simulink library "simetranss"  (R2024b)
settings: Solver=VariableStepAuto  StartTime=0.0  StopTime=10.0  RelTol=1e-3
PostLoadFcn:
  | Ts=1e-6
InitFcn:
  | Ts=1e-6
undefined symbols (not defined in the file): C, C_601, C_603, C_606, CC, Csnu, Csnubber, DiscIntNeverNeededParam, DPL, DPL1ph, FluxTable, ft2km, gcbh, h, Half, Imap2, L, L_601, L_603, L_606, Lbase, LpejoSw, Newton, R_601, R_603, R_606, Raphson, ResistanceM, Roff, Ron, RotorAngles, Rsnu, Rsnubber, Rt4, SampleTime, simetran, sps, sps_rtmsupport, StatorCurrents, T_2wind_ratio, T_Lpu, T_Lpu_pri, T_Rpu, T_Rpu_pri, T_Vpri, T_Vpri_15comp, T_Vsec, Ti, Ts_Power, Z, Zbase, Zm
libraries: fl_lib x248, ee_lib x146, nesl_utility x122, $bdroot x29, simulink x15, eeGeneralControl x2, spsStairGeneratorLib x2, artemis x1
(part 8 of 12)

== system simetranss/Power converters/Switching Function Interpolating 2-level inverter ==
  g : Inport
  Constant1 : Constant  Value=0
  Constant9 : Constant  Value=0
  Controlled Current Source1 : fl_lib/Electrical/Electrical Sources/Controlled Current Source
  Controlled Voltage Source : fl_lib/Electrical/Electrical Sources/Controlled Voltage Source
  Current Sensor : fl_lib/Electrical/Electrical Sensors/Current Sensor
  Demux1 : Demux  Outputs=2
  Fcn : Fcn  Expr=1-u
  PS-Simulink Converter : nesl_utility/PS-Simulink Converter  PhysicalDomain=network_engine_domain  SubClassName=ps_output  LeftPortType=input  RightPortType=output  PseudoPeriodic=off  Frequencies=[]  VectorFormat=inherit  Unit=inherit  AffineConversion=off
  PS-Simulink Converter1 : nesl_utility/PS-Simulink Converter  PhysicalDomain=network_engine_domain  SubClassName=ps_output  LeftPortType=input  RightPortType=output  PseudoPeriodic=off  Frequencies=[]  VectorFormat=inherit  Unit=inherit  AffineConversion=off
  Simulink-PS Converter : nesl_utility/Simulink-PS Converter  PhysicalDomain=network_engine_domain  SubClassName=ps_input  LeftPortType=input  RightPortType=output  PseudoPeriodic=off  Frequencies=[]  NoiseDistribution=none  NoiseParameters=[]  Unit=1  AffineConversion=off  FilteringAndDerivatives=provide  SimscapeFilterOrder=1  InputFilterTimeConstant=0.001  UdotUserProvided=0
  Simulink-PS Converter1 : nesl_utility/Simulink-PS Converter  PhysicalDomain=network_engine_domain  SubClassName=ps_input  LeftPortType=input  RightPortType=output  PseudoPeriodic=off  Frequencies=[]  NoiseDistribution=none  NoiseParameters=[]  Unit=1  AffineConversion=off  FilteringAndDerivatives=provide  SimscapeFilterOrder=1  InputFilterTimeConstant=0.001  UdotUserProvided=0
  Simulink-PS Converter2 : nesl_utility/Simulink-PS Converter  PhysicalDomain=network_engine_domain  SubClassName=ps_input  LeftPortType=input  RightPortType=output  PseudoPeriodic=off  Frequencies=[]  NoiseDistribution=none  NoiseParameters=[]  Unit=1  AffineConversion=off  FilteringAndDerivatives=provide  SimscapeFilterOrder=1  InputFilterTimeConstant=0.001  UdotUserProvided=0
  Switch : fl_lib/Electrical/Electrical Elements/Switch  R_closed=Ron Ohm  G_open=1e-5 1/Ohm  Threshold=0.5  i_specify=off  i_priority=None  i=0 A  i_nominal_specify=off  i_nominal_value=1  i_nominal_unit=A  v_specify=off  v_priority=None  v=0 V  v_nominal_specify=off  v_nominal_value=1  v_nominal_unit=V
  Switch1 : Switch  Threshold=0.5  SaturateOnIntegerOverflow=off  InputSameDT=off
  Switch4 : Switch  Threshold=0.5  SaturateOnIntegerOverflow=off  InputSameDT=off
  Unit Delay : UnitDelay  SampleTime=Ts  HasFrameUpgradeWarning=on
  Unit Delay1 : UnitDelay  SampleTime=Ts  HasFrameUpgradeWarning=on
  Voltage Sensor : fl_lib/Electrical/Electrical Sensors/Voltage Sensor
  ctrl1 : Subsystem
  lowthy : Subsystem
  upthy : Subsystem
  A : PMIOPort  Side=Left
  Dc+ : PMIOPort  Port=2  Side=Right
  Dc- : PMIOPort  Port=3  Side=Right
  wires:
  ctrl1/3(sw) -> [sw], Switch4/2, Switch1/2
  ctrl1/1(Idc) -> Switch1/1
  Switch1/1 -> Simulink-PS Converter/1
  Constant1/1 -> Switch1/3
  ctrl1/2(Vac) -> Switch4/1
  Constant9/1 -> Switch4/3
  Switch4/1 -> Simulink-PS Converter1/1
  Unit Delay1/1 -> ctrl1/3(Iac)
  Unit Delay/1 -> ctrl1/4(Vdc)
  Fcn/1 -> upthy/1(g), lowthy/1(g)
  [sw] -> Fcn/1
  [sw] -> Simulink-PS Converter2/1
  PS-Simulink Converter1/1 -> Unit Delay/1
  PS-Simulink Converter/1 -> lowthy/2(i), upthy/2("i "), Unit Delay1/1
  Demux1/1 -> ctrl1/1(g)
  Demux1/2 -> ctrl1/2(g1)
  g/1 -> Demux1/1
  connections:
  Switch/LConn1 -- Current Sensor/LConn1
  Controlled Voltage Source/LConn1 -- Switch/RConn2
  Current Sensor/RConn2 -- lowthy/RConn1 -- upthy/LConn1 -- A/RConn1
  PS-Simulink Converter1/LConn1 -- Voltage Sensor/RConn1
  upthy/RConn1 -- Dc+/RConn1 -- Voltage Sensor/LConn1 -- Controlled Current Source1/RConn2
  lowthy/LConn1 -- Voltage Sensor/RConn2 -- Controlled Voltage Source/RConn2 -- Controlled Current Source1/LConn1 -- Dc-/RConn1
  Simulink-PS Converter1/RConn1 -- Controlled Voltage Source/RConn1
  PS-Simulink Converter/LConn1 -- Current Sensor/RConn1
  Simulink-PS Converter/RConn1 -- Controlled Current Source1/RConn1
  Simulink-PS Converter2/RConn1 -- Switch/RConn1

== system simetranss/Switches/MATE 3ph Breaker ==
  C4 : Constant  Value=External
  Circuit Breaker : ee_lib/Switches & Breakers/Circuit Breaker  R_closed=BreakerResistance Ohm  G_open=1/Roff 1/Ohm  threshold=0.5 V  breaker_behavior=ee.enum.switches.breakerBehavior.zeroCrossingEnable
      settings: InternalSimscapePortConfiguration="{\"Bottom\":[],\"Left\":[{\"id\":\"vT\",\"label\":\"vT\",\"type\":\"input\"},{\"id\":\"p1\",\"label\":\"\",\"type\":\"foundation.electrical.electrical\"}],\"Right\":[{\"id\":\"p2\",\"label\":\"\",\"type\":\"foundation.electrical.electrical\"}],\"Top\":[]}"
  Circuit Breaker1 : ee_lib/Switches & Breakers/Circuit Breaker  R_closed=BreakerResistance Ohm  G_open=1/Roff 1/Ohm  threshold=0.5 V  breaker_behavior=ee.enum.switches.breakerBehavior.zeroCrossingEnable
      settings: InternalSimscapePortConfiguration="{\"Bottom\":[],\"Left\":[{\"id\":\"vT\",\"label\":\"vT\",\"type\":\"input\"},{\"id\":\"p1\",\"label\":\"\",\"type\":\"foundation.electrical.electrical\"}],\"Right\":[{\"id\":\"p2\",\"label\":\"\",\"type\":\"foundation.electrical.electrical\"}],\"Top\":[]}"
  Circuit Breaker2 : ee_lib/Switches & Breakers/Circuit Breaker  R_closed=BreakerResistance Ohm  G_open=1/Roff 1/Ohm  threshold=0.5 V  breaker_behavior=ee.enum.switches.breakerBehavior.zeroCrossingEnable
      settings: InternalSimscapePortConfiguration="{\"Bottom\":[],\"Left\":[{\"id\":\"vT\",\"label\":\"vT\",\"type\":\"input\"},{\"id\":\"p1\",\"label\":\"\",\"type\":\"foundation.electrical.electrical\"}],\"Right\":[{\"id\":\"p2\",\"label\":\"\",\"type\":\"foundation.electrical.electrical\"}],\"Top\":[]}"
  Constant1 : Constant  Value=SwitchA
  Constant2 : Constant  Value=SwitchB
  Constant3 : Constant  Value=SwitchC
  Constant5 : Constant  Value=InitialState
  Fcn : Fcn  Expr=1-u
  Fcn1 : Fcn  Expr=1-u
  Fcn2 : Fcn  Expr=1-u
  Phase Splitter1 : ee_lib/Connectors & References/Phase Splitter
  Phase Splitter2 : ee_lib/Connectors & References/Phase Splitter
  RCsnubber : Subsystem  Commented=on
  Simulink-PS Converter : nesl_utility/Simulink-PS Converter  PhysicalDomain=network_engine_domain  SubClassName=ps_input  LeftPortType=input  RightPortType=output  PseudoPeriodic=off  Frequencies=[]  NoiseDistribution=none  NoiseParameters=[]  Unit=1  AffineConversion=off  FilteringAndDerivatives=provide  SimscapeFilterOrder=1  InputFilterTimeConstant=0.001  UdotUserProvided=0
  Simulink-PS Converter1 : nesl_utility/Simulink-PS Converter  PhysicalDomain=network_engine_domain  SubClassName=ps_input  LeftPortType=input  RightPortType=output  PseudoPeriodic=off  Frequencies=[]  NoiseDistribution=none  NoiseParameters=[]  Unit=1  AffineConversion=off  FilteringAndDerivatives=provide  SimscapeFilterOrder=1  InputFilterTimeConstant=0.001  UdotUserProvided=0
  Simulink-PS Converter2 : nesl_utility/Simulink-PS Converter  PhysicalDomain=network_engine_domain  SubClassName=ps_input  LeftPortType=input  RightPortType=output  PseudoPeriodic=off  Frequencies=[]  NoiseDistribution=none  NoiseParameters=[]  Unit=1  AffineConversion=off  FilteringAndDerivatives=provide  SimscapeFilterOrder=1  InputFilterTimeConstant=0.001  UdotUserProvided=0
  Stair Generator : spsStairGeneratorLib/Stair Generator  t=Switch_Times  e=SwitchStates  Ts=Ts
  Switch : Switch  Threshold=0.5  ZeroCross=off  SaturateOnIntegerOverflow=off
  Switch1 : Switch  Threshold=0.5  ZeroCross=off  SaturateOnIntegerOverflow=off
  Switch2 : Switch  Threshold=0.5  ZeroCross=off  SaturateOnIntegerOverflow=off
  Switch3 : Switch  Threshold=0.5  ZeroCross=off  SaturateOnIntegerOverflow=off  InputSameDT=off
  com : Constant
  abc : PMIOPort  Side=Left
  ABC : PMIOPort  Port=2  Side=Right
  wires:
  Switch3/1 -> Switch2/1, Switch1/1, Switch/1
  Constant1/1 -> Switch/2
  Switch/1 -> Fcn/1
  Constant3/1 -> Switch2/2
  Switch2/1 -> Fcn2/1
  Constant2/1 -> Switch1/2
  Switch1/1 -> Fcn1/1
  C4/1 -> Switch3/2
  com/1 -> Switch3/1
  Stair Generator/1 -> Switch3/3
  Constant5/1 -> Switch/3, Switch1/3, Switch2/3
  Fcn/1 -> Simulink-PS Converter/1
  Fcn1/1 -> Simulink-PS Converter1/1
  Fcn2/1 -> Simulink-PS Converter2/1
  connections:
  Circuit Breaker/LConn1 -- Simulink-PS Converter/RConn1
  RCsnubber/LConn2 -- Phase Splitter2/RConn2 -- Circuit Breaker1/LConn2
  Phase Splitter2/LConn1 -- abc/RConn1
  Circuit Breaker/LConn2 -- Phase Splitter2/RConn1 -- RCsnubber/LConn3
  RCsnubber/LConn1 -- Phase Splitter2/RConn3 -- Circuit Breaker2/LConn2
  Circuit Breaker1/LConn1 -- Simulink-PS Converter1/RConn1
  Circuit Breaker2/LConn1 -- Simulink-PS Converter2/RConn1
  Phase Splitter1/LConn1 -- ABC/RConn1
  Phase Splitter1/RConn1 -- Circuit Breaker/RConn1 -- RCsnubber/RConn1
  RCsnubber/RConn2 -- Phase Splitter1/RConn2 -- Circuit Breaker1/RConn1
  RCsnubber/RConn3 -- Phase Splitter1/RConn3 -- Circuit Breaker2/RConn1

== system simetranss/Switches/MATE Breaker ==
  C4 : Constant  Value=External
  Circuit Breaker : ee_lib/Switches & Breakers/Circuit Breaker  R_closed=BreakerResistance Ohm  G_open=1/Roff 1/Ohm  threshold=0.5 V  breaker_behavior=ee.enum.switches.breakerBehavior.zeroCrossingEnable
      settings: InternalSimscapePortConfiguration="{\"Bottom\":[],\"Left\":[{\"id\":\"vT\",\"label\":\"vT\",\"type\":\"input\"},{\"id\":\"p1\",\"label\":\"\",\"type\":\"foundation.electrical.electrical\"}],\"Right\":[{\"id\":\"p2\",\"label\":\"\",\"type\":\"foundation.electrical.electrical\"}],\"Top\":[]}"
  Constant1 : Constant  Value=SwitchA
  Constant5 : Constant  Value=InitialState
  Fcn : Fcn  Expr=1-u
  RCsnubber : Subsystem  Commented=on
  Simulink-PS Converter : nesl_utility/Simulink-PS Converter  PhysicalDomain=network_engine_domain  SubClassName=ps_input  LeftPortType=input  RightPortType=output  PseudoPeriodic=off  Frequencies=[]  NoiseDistribution=none  NoiseParameters=[]  Unit=1  AffineConversion=off  FilteringAndDerivatives=provide  SimscapeFilterOrder=1  InputFilterTimeConstant=0.001  UdotUserProvided=0
  Stair Generator : spsStairGeneratorLib/Stair Generator  t=Switch_Times  e=SwitchStates  Ts=Ts
  Switch : Switch  Threshold=0.5  ZeroCross=off  SaturateOnIntegerOverflow=off
  Switch3 : Switch  Threshold=0.5  ZeroCross=off  SaturateOnIntegerOverflow=off  InputSameDT=off
  com : Constant
  a : PMIOPort  Side=Left
  A : PMIOPort  Port=2  Side=Right
  wires:
  Fcn/1 -> Simulink-PS Converter/1
  Constant5/1 -> Switch/3
  Stair Generator/1 -> Switch3/3
  com/1 -> Switch3/1
  C4/1 -> Switch3/2
  Switch/1 -> Fcn/1
  Constant1/1 -> Switch/2
  Switch3/1 -> Switch/1
  connections:
  Circuit Breaker/RConn1 -- RCsnubber/RConn1 -- A/RConn1
  Circuit Breaker/LConn2 -- RCsnubber/LConn1 -- a/RConn1
  Circuit Breaker/LConn1 -- Simulink-PS Converter/RConn1

== system simetranss/Usefulls/Event Timer ==
  Repeating Sequence : simulink/Sources/Repeating Sequence  rep_seq_t=st  rep_seq_y=sw
  Repeating Sequence1 : simulink/Sources/Repeating Sequence  Commented=on  rep_seq_t="[0    0.2000    0.2001    0.4000    0.4001    0.6000    2.0000]"  rep_seq_y=|
      | [     1     1     0     0     1     1     1
      | ]
  RTE : Outport  VectorParamsAs1DForOutWhenUnconnected=off
  wires:
  Repeating Sequence/1 -> RTE/1

== system simetranss/Usefulls/ModelInitialization ==

== system simetranss/FPGA/MATE 2-level inverter backup/Pejovic L//C switch2 ==
  gate : Inport
  Xin : Inport  Port=2
  Bus Creator : BusCreator  Inputs=2
  Controlled Current Source : fl_lib/Electrical/Electrical Sources/Controlled Current Source
  Current Sensor : fl_lib/Electrical/Electrical Sensors/Current Sensor
  Gain : Gain  Gain=-1
  Gain1 : Gain  Gain=1/Rsw
  Gain2 : Gain
  PS-Simulink Converter1 : nesl_utility/PS-Simulink Converter  PhysicalDomain=network_engine_domain  SubClassName=ps_output  LeftPortType=input  RightPortType=output  PseudoPeriodic=off  Frequencies=[]  VectorFormat=inherit  Unit=inherit  AffineConversion=off
  PS-Simulink Converter2 : nesl_utility/PS-Simulink Converter  PhysicalDomain=network_engine_domain  SubClassName=ps_output  LeftPortType=input  RightPortType=output  PseudoPeriodic=off  Frequencies=[]  VectorFormat=inherit  Unit=inherit  AffineConversion=off
  Relational Operator : RelationalOperator  Operator=~=  OutDataTypeStr=boolean  RndMeth=Simplest  InputSameDT=off
  Resistor : fl_lib/Electrical/Electrical Elements/Resistor  R=Rsw Ohm  i_specify=off  i_priority=None  i=0 A  i_nominal_specify=off  i_nominal_value=1  i_nominal_unit=A  v_specify=off  v_priority=None  v=0 V  v_nominal_specify=off  v_nominal_value=1  v_nominal_unit=V
  Simulink-PS Converter1 : nesl_utility/Simulink-PS Converter  PhysicalDomain=network_engine_domain  SubClassName=ps_input  LeftPortType=input  RightPortType=output  PseudoPeriodic=off  Frequencies=[]  NoiseDistribution=none  NoiseParameters=[]  Unit=1  AffineConversion=off  FilteringAndDerivatives=provide  SimscapeFilterOrder=1  InputFilterTimeConstant=0.001  UdotUserProvided=0
  Switch : Switch  Criteria=u2 > Threshold  Threshold=0.5  SaturateOnIntegerOverflow=off  InputSameDT=off
  Switch1 : Switch  Criteria=u2 > Threshold  Threshold=0.5  SaturateOnIntegerOverflow=off  InputSameDT=off
  Switch2 : Switch  Criteria=u2 > Threshold  Threshold=0.5  SaturateOnIntegerOverflow=off  InputSameDT=off
  Unit Delay : UnitDelay  SampleTime=Ts  HasFrameUpgradeWarning=on
  Unit Delay1 : UnitDelay  SampleTime=Ts  HasFrameUpgradeWarning=on
  Unit Delay2 : UnitDelay  SampleTime=Ts  HasFrameUpgradeWarning=on
  Voltage Sensor : fl_lib/Electrical/Electrical Sensors/Voltage Sensor
  +V : PMIOPort  Side=Left
  -V : PMIOPort  Port=2  Side=Right
  meas : Outport
  Xout : Outport  Port=2
  wires:
  PS-Simulink Converter2/1 -> [Vsw]
  PS-Simulink Converter1/1 -> [Isw]
  Switch/1 -> Unit Delay/1
  [Isw] -> Gain/1
  Gain/1 -> Switch/1
  [Vsw] -> Gain1/1
  Gain1/1 -> Switch2/3, Switch/3
  [Ihist] -> Simulink-PS Converter1/1
  [Isw] -> Bus Creator/2  "Switch current (A)"
  [Vsw] -> Bus Creator/1  "Switch voltage (V)"
  Bus Creator/1 -> meas/1
  Switch1/1 -> [Ihist]
  Unit Delay/1 -> Switch1/3
  Xin/1 -> Switch1/1
  Unit Delay1/1 -> Relational Operator/1
  Relational Operator/1 -> Switch1/2
  Gain2/1 -> Switch2/1
  [Isw] -> Gain2/1
  Switch2/1 -> Unit Delay2/1
  gate/1 -> Switch2/2, Relational Operator/2, Unit Delay1/1, Switch/2
  Unit Delay2/1 -> Xout/1
  connections:
  Resistor/RConn1 -- Voltage Sensor/RConn2 -- -V/RConn1 -- Controlled Current Source/RConn2
  Current Sensor/RConn2 -- Voltage Sensor/LConn1 -- Resistor/LConn1 -- Controlled Current Source/LConn1
  PS-Simulink Converter2/LConn1 -- Voltage Sensor/RConn1
  Controlled Current Source/RConn1 -- Simulink-PS Converter1/RConn1
  +V/RConn1 -- Current Sensor/LConn1
  Current Sensor/RConn1 -- PS-Simulink Converter1/LConn1

== system simetranss/FPGA/MATE 2-level inverter backup/Pejovic L//C switch3 ==
  gate : Inport
  Xin : Inport  Port=2
  Bus Creator : BusCreator  Inputs=2
  Controlled Current Source : fl_lib/Electrical/Electrical Sources/Controlled Current Source
  Current Sensor : fl_lib/Electrical/Electrical Sensors/Current Sensor
  Gain : Gain  Gain=-1
  Gain1 : Gain  Gain=1/Rsw
  Gain2 : Gain
  PS-Simulink Converter1 : nesl_utility/PS-Simulink Converter  PhysicalDomain=network_engine_domain  SubClassName=ps_output  LeftPortType=input  RightPortType=output  PseudoPeriodic=off  Frequencies=[]  VectorFormat=inherit  Unit=inherit  AffineConversion=off
  PS-Simulink Converter2 : nesl_utility/PS-Simulink Converter  PhysicalDomain=network_engine_domain  SubClassName=ps_output  LeftPortType=input  RightPortType=output  PseudoPeriodic=off  Frequencies=[]  VectorFormat=inherit  Unit=inherit  AffineConversion=off
  Relational Operator : RelationalOperator  Operator=~=  OutDataTypeStr=boolean  RndMeth=Simplest  InputSameDT=off
  Resistor : fl_lib/Electrical/Electrical Elements/Resistor  R=Rsw Ohm  i_specify=off  i_priority=None  i=0 A  i_nominal_specify=off  i_nominal_value=1  i_nominal_unit=A  v_specify=off  v_priority=None  v=0 V  v_nominal_specify=off  v_nominal_value=1  v_nominal_unit=V
  Simulink-PS Converter1 : nesl_utility/Simulink-PS Converter  PhysicalDomain=network_engine_domain  SubClassName=ps_input  LeftPortType=input  RightPortType=output  PseudoPeriodic=off  Frequencies=[]  NoiseDistribution=none  NoiseParameters=[]  Unit=1  AffineConversion=off  FilteringAndDerivatives=provide  SimscapeFilterOrder=1  InputFilterTimeConstant=0.001  UdotUserProvided=0
  Switch : Switch  Criteria=u2 > Threshold  Threshold=0.5  SaturateOnIntegerOverflow=off  InputSameDT=off
  Switch1 : Switch  Criteria=u2 > Threshold  Threshold=0.5  SaturateOnIntegerOverflow=off  InputSameDT=off
  Switch2 : Switch  Criteria=u2 > Threshold  Threshold=0.5  SaturateOnIntegerOverflow=off  InputSameDT=off
  Unit Delay : UnitDelay  SampleTime=Ts  HasFrameUpgradeWarning=on
  Unit Delay1 : UnitDelay  SampleTime=Ts  HasFrameUpgradeWarning=on
  Unit Delay2 : UnitDelay  SampleTime=Ts  HasFrameUpgradeWarning=on
  Voltage Sensor : fl_lib/Electrical/Electrical Sensors/Voltage Sensor
  +V : PMIOPort  Side=Left
  -V : PMIOPort  Port=2  Side=Right
  meas : Outport
  Xout : Outport  Port=2
  wires:
  Relational Operator/1 -> Switch1/2
  Unit Delay1/1 -> Relational Operator/1
  Xin/1 -> Switch1/1
  Unit Delay/1 -> Switch1/3
  Switch1/1 -> [Ihist]
  Bus Creator/1 -> meas/1
  [Vsw] -> Bus Creator/1  "Switch voltage (V)"
  [Isw] -> Bus Creator/2  "Switch current (A)"
  [Ihist] -> Simulink-PS Converter1/1
  [Vsw] -> Gain1/1
  Gain/1 -> Switch/1
  [Isw] -> Gain/1
  Switch/1 -> Unit Delay/1
  PS-Simulink Converter1/1 -> [Isw]
  PS-Simulink Converter2/1 -> [Vsw]
  Gain2/1 -> Switch2/1
  [Isw] -> Gain2/1
  gate/1 -> Switch/2, Switch2/2, Unit Delay1/1, Relational Operator/2
  Switch2/1 -> Unit Delay2/1
  Gain1/1 -> Switch/3, Switch2/3
  Unit Delay2/1 -> Xout/1
  connections:
  Current Sensor/RConn1 -- PS-Simulink Converter1/LConn1
  +V/RConn1 -- Current Sensor/LConn1
  Controlled Current Source/RConn1 -- Simulink-PS Converter1/RConn1
  PS-Simulink Converter2/LConn1 -- Voltage Sensor/RConn1
  Controlled Current Source/LConn1 -- Resistor/LConn1 -- Voltage Sensor/LConn1 -- Current Sensor/RConn2
  Controlled Current Source/RConn2 -- -V/RConn1 -- Voltage Sensor/RConn2 -- Resistor/RConn1

== system simetranss/FPGA/MATE 2level_Inverter SwitchingFunction(3ph)/SW ==
  note: 1 = no pulse
      | 0 = pulse
  note: 0 == mode diode
      | 0 ~= mode pulse
  note: 1 = mode HighZ
      | 0 = mode pulse or diode
  gu : Inport
  gl : Inport  Port=2
  Vdc : Inport  Port=3
  Iac : Inport  Port=4
  Compare To Zero : simulink/Logic and Bit Operations/Compare To Zero  relop=>  OutDataTypeStr=uint8
  Constant : Constant
  Dead Zone : DeadZone  LowerValue=-min_charge  UpperValue=min_charge
  Divide : Product  Inputs=3
  Divide1 : Product
  Divide3 : Product
  Gain1 : Gain  Gain=Gp
  INT : Subsystem
  Logical Operator{1,4..5,8} (4 alike) : Logic  AllPortsSameDT=off  OutDataTypeStr=boolean
  Logical Operator{2..3,7,9} (4 alike) : Logic  Operator=NOT  AllPortsSameDT=off  OutDataTypeStr=boolean
  Logical Operator6 : Logic  Operator=OR  Inputs=3  AllPortsSameDT=off  OutDataTypeStr=boolean
  Logical_Not1 : Constant  Value=0  SampleTime=-1
  Relational Operator1 : RelationalOperator  Operator=>  OutDataTypeStr=boolean  InputSameDT=off
  Sum : Sum  Inputs=|++
  Sum1 : Sum  Inputs=--+
  Sum2 : Sum  Inputs=|++
  Sum6 : Sum  Inputs=-+  InputSameDT=on  SaturateOnIntegerOverflow=on  SampleTime=Ts  OutDataTypeStr=Inherit: Same as first input
  Switch : Switch  Criteria=u2 > Threshold  SaturateOnIntegerOverflow=off  InputSameDT=off
  Switch1 : Switch  Criteria=u2 ~= 0  SaturateOnIntegerOverflow=off  InputSameDT=off
  Switch2 : Switch  Criteria=u2 ~= 0  Threshold=0.5  SaturateOnIntegerOverflow=off  InputSameDT=off
  Switch3 : Switch  Criteria=u2 ~= 0  Threshold=0.5  SaturateOnIntegerOverflow=off  InputSameDT=off
  Unit Delay1 : UnitDelay  SampleTime=Ts  HasFrameUpgradeWarning=on
  Unit Delay2 : UnitDelay  SampleTime=Ts  HasFrameUpgradeWarning=on
  Idc : Outport  VectorParamsAs1DForOutWhenUnconnected=off
  Vac : Outport  Port=2  VectorParamsAs1DForOutWhenUnconnected=off
  wires:
  Unit Delay2/1 -> Logical Operator8/2, Logical Operator9/1
  Unit Delay1/1 -> [Vout]
  Switch3/1 -> Switch2/3
  Dead Zone/1 -> Switch3/1
  Divide/1 -> Dead Zone/1, Switch2/1, Switch3/3
  Switch2/1 -> Idc/1
  Switch/1 -> Switch1/1
  Logical Operator6/1 -> Logical Operator1/2, Unit Delay2/1
  Divide1/1 -> Switch1/3
  Sum2/1 -> Divide/2, Divide1/2
  gu/1 -> Sum1/1, Sum2/1, Sum/1
  Sum/1 -> Logical Operator2/1
  Compare To Zero/1 -> Logical Operator5/1, Logical Operator4/1, Logical Operator7/1
  Vdc/1 -> [Vin], Divide1/1
  [Vout] -> Relational Operator1/2
  Logical Operator2/1 -> Logical Operator1/1, Switch3/2
  Logical Operator3/1 -> Divide/3
  [Vin] -> Relational Operator1/1
  gl/1 -> Sum/2, Sum1/2
  Logical Operator7/1 -> Divide3/1
  Relational Operator1/1 -> Logical Operator5/2, Logical Operator8/1
  Logical Operator9/1 -> Logical Operator4/2
  Logical Operator4/1 -> Logical Operator6/1
  Logical Operator5/1 -> Logical Operator6/2
  Logical Operator8/1 -> Logical Operator6/3
  Constant/1 -> Sum1/3
  Sum1/1 -> Divide3/2
  Divide3/1 -> Sum2/2
  Switch1/1 -> Vac/1, Unit Delay1/1
  [Vout] -> INT/2(Initial)
  INT/1(u_p) -> Sum6/2
  Sum6/1 -> Switch/2, Switch/1
  Logical_Not1/1 -> Switch/3
  Logical Operator1/1 -> Switch2/2, Switch1/2, INT/3(en), Logical Operator3/1
  Gain1/1 -> Sum6/1
  Iac/1 -> Divide/1, Compare To Zero/1, INT/1(u), Gain1/1

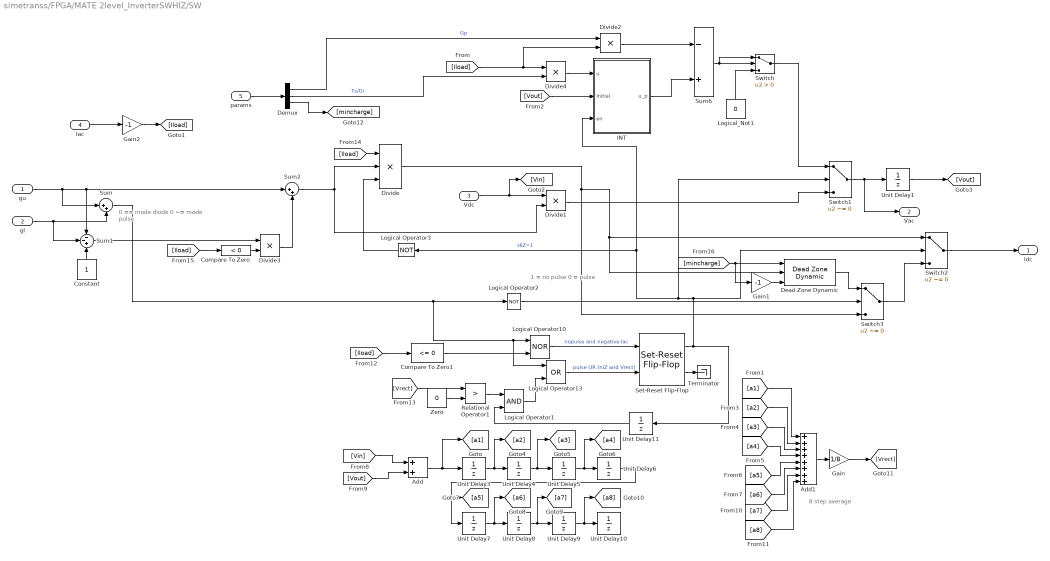
== system simetranss/FPGA/MATE 2level_InverterSWHIZ/SW ==
  note: 8 step average
  note: 1 = no pulse
      | 0 = pulse
  note: 0 == mode diode
      | 0 ~= mode pulse
  gu : Inport
  gl : Inport  Port=2
  Vdc : Inport  Port=3
  Iac : Inport  Port=4
  params : Inport  Port=5
  Add : Sum
  Add1 : Sum  Inputs=8
  Compare To Zero : simulink/Logic and Bit Operations/Compare To Zero  relop=<  OutDataTypeStr=uint8
  Compare To Zero1 : simulink/Logic and Bit Operations/Compare To Zero  relop=<=  OutDataTypeStr=uint8
  Constant : Constant
  Dead Zone Dynamic : simulink/Discontinuities/Dead Zone Dynamic
  Demux : Demux  Outputs=3
  Divide : Product  Inputs=3
  Divide{1..4} (4 alike) : Product
  Gain : Gain  Gain=1/8
  Gain1 : Gain  Gain=-1
  Gain2 : Gain  Gain=-1
  INT : Subsystem
  Logical Operator1 : Logic  AllPortsSameDT=off  OutDataTypeStr=boolean
  Logical Operator10 : Logic  Operator=NOR  AllPortsSameDT=off  OutDataTypeStr=boolean
  Logical Operator13 : Logic  Operator=OR  AllPortsSameDT=off  OutDataTypeStr=boolean
  Logical Operator2 : Logic  Operator=NOT  AllPortsSameDT=off  OutDataTypeStr=boolean
  Logical Operator3 : Logic  Operator=NOT  AllPortsSameDT=off  OutDataTypeStr=boolean
  Logical_Not1 : Constant  Value=0  SampleTime=-1
  Relational Operator1 : RelationalOperator  Operator=>  OutDataTypeStr=boolean  InputSameDT=off
  Set-Reset Flip-Flop : eeGeneralControl/Set-Reset Flip-Flop  LabelModeActiveChoice=Discrete  UndefState=Set  Q0=0  Ts=Ts
  Sum : Sum  Inputs=|++
  Sum1 : Sum  Inputs=--+
  Sum2 : Sum  Inputs=|++
  Sum6 : Sum  Inputs=-+  InputSameDT=on  SaturateOnIntegerOverflow=on  SampleTime=Ts  OutDataTypeStr=Inherit: Same as first input
  Switch : Switch  Criteria=u2 > Threshold  SaturateOnIntegerOverflow=off  InputSameDT=off
  Switch1 : Switch  Criteria=u2 ~= 0  SaturateOnIntegerOverflow=off  InputSameDT=off
  Switch2 : Switch  Criteria=u2 ~= 0  Threshold=0.5  SaturateOnIntegerOverflow=off  InputSameDT=off
  Switch3 : Switch  Criteria=u2 ~= 0  Threshold=0.5  SaturateOnIntegerOverflow=off  InputSameDT=off
  Terminator : Terminator
  Unit Delay{1,3..11} (10 alike) : UnitDelay  SampleTime=Ts  HasFrameUpgradeWarning=on
  Zero : Constant  Value=0  OutDataTypeStr=Inherit: Inherit via back propagation
  Idc : Outport  VectorParamsAs1DForOutWhenUnconnected=off
  Vac : Outport  Port=2  VectorParamsAs1DForOutWhenUnconnected=off
  wires:
  params/1 -> Demux/1
  Gain1/1 -> Dead Zone Dynamic/3
  [mincharge] -> Gain1/1, Dead Zone Dynamic/1
  Demux/3 -> [mincharge]
  Demux/2 -> Divide4/2  "Ts/Gi"
  Divide4/1 -> INT/1(u)
  Divide2/1 -> Sum6/1
  Demux/1 -> Divide2/1  "Gp"
  Gain2/1 -> [Iload]
  Sum1/1 -> Divide3/1
  Compare To Zero/1 -> Divide3/2
  [Iload] -> Compare To Zero/1
  [Iload] -> Divide/1
  [Iload] -> Divide2/2, Divide4/1
  Logical Operator1/1 -> Logical Operator13/2
  Logical Operator13/1 -> Set-Reset Flip-Flop/2  "pulse OR (hiZ and Vrect)"
  Unit Delay11/1 -> Logical Operator1/2
  Relational Operator1/1 -> Logical Operator1/1
  Zero/1 -> Relational Operator1/2
  [Vrect] -> Relational Operator1/1
  INT/1(u_p) -> Sum6/2
  Compare To Zero1/1 -> Logical Operator10/2
  [Iload] -> Compare To Zero1/1
  Gain/1 -> [Vrect]
  Add1/1 -> Gain/1
  [a1] -> Add1/1
  [a8] -> Add1/8
  [a2] -> Add1/2
  [a7] -> Add1/7
  [a6] -> Add1/6
  [a3] -> Add1/3
  [a5] -> Add1/5
  [a4] -> Add1/4
  Unit Delay9/1 -> Unit Delay10/1, [a8]
  Unit Delay8/1 -> Unit Delay9/1, [a7]
  Unit Delay7/1 -> Unit Delay8/1, [a6]
  Unit Delay6/1 -> Unit Delay7/1, [a5]
  Unit Delay5/1 -> Unit Delay6/1, [a4]
  Unit Delay4/1 -> Unit Delay5/1, [a3]
  Unit Delay3/1 -> Unit Delay4/1, [a2]
  Add/1 -> Unit Delay3/1, [a1]
  [Vout] -> Add/2
  [Vin] -> Add/1
  [Vout] -> INT/2(Initial)
  Logical Operator10/1 -> Set-Reset Flip-Flop/1  "nopulse and negative Iac"
  Unit Delay1/1 -> [Vout]
  Switch3/1 -> Switch2/3
  Dead Zone Dynamic/1 -> Switch3/1
  Divide/1 -> Switch2/1, Dead Zone Dynamic/2, Switch3/3
  Switch2/1 -> Idc/1
  Switch/1 -> Switch1/1
  Divide1/1 -> Switch1/3
  Sum2/1 -> Divide/2, Divide1/2
  gu/1 -> Sum1/1, Sum2/1, Sum/1
  Sum/1 -> Logical Operator2/1, Logical Operator10/1, Logical Operator13/1
  Vdc/1 -> [Vin], Divide1/1
  Logical Operator2/1 -> Switch3/2
  Logical Operator3/1 -> Divide/3
  gl/1 -> Sum/2, Sum1/2
  Constant/1 -> Sum1/3
  Divide3/1 -> Sum2/2
  Switch1/1 -> Vac/1, Unit Delay1/1
  Sum6/1 -> Switch/2, Switch/1
  Logical_Not1/1 -> Switch/3
  Set-Reset Flip-Flop/1 -> Unit Delay11/1, Switch2/2, Switch1/2, INT/3(en), Logical Operator3/1  "HiZ=1"
  Iac/1 -> Gain2/1
  Set-Reset Flip-Flop/2 -> Terminator/1

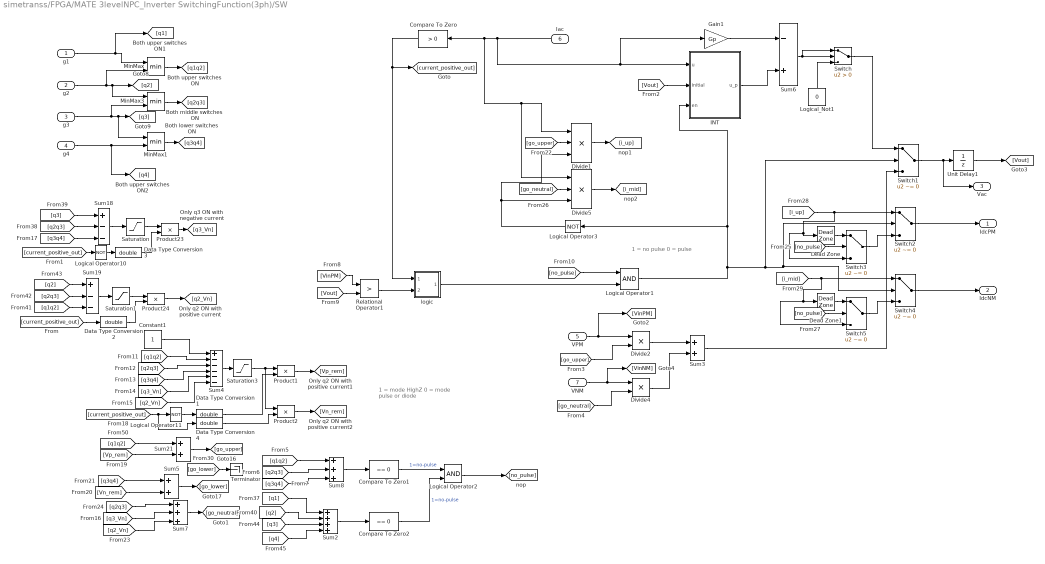
== system simetranss/FPGA/MATE 3levelNPC_Inverter SwitchingFunction(3ph)/SW ==
  note: 1 = no pulse
      | 0 = pulse
  note: 1 = mode HighZ
      | 0 = mode pulse or diode
  g1 : Inport
  g2 : Inport  Port=2
  g3 : Inport  Port=3
  g4 : Inport  Port=4
  VPM : Inport  Port=5
  Iac : Inport  Port=6
  VNM : Inport  Port=7
  Compare To Zero : simulink/Logic and Bit Operations/Compare To Zero  relop=>  OutDataTypeStr=uint8
  Compare To Zero1 : simulink/Logic and Bit Operations/Compare To Zero  relop===  OutDataTypeStr=uint8
  Compare To Zero2 : simulink/Logic and Bit Operations/Compare To Zero  relop===  OutDataTypeStr=uint8
  Constant1 : Constant
  Data Type Conversion{1..4} (4 alike) : DataTypeConversion  OutDataTypeStr=double
  Dead Zone : DeadZone  LowerValue=-min_charge  UpperValue=min_charge
  Dead Zone1 : DeadZone  LowerValue=-min_charge  UpperValue=min_charge
  Divide1 : Product  Inputs=3
  Divide2 : Product
  Divide4 : Product
  Divide5 : Product  Inputs=3
  Gain1 : Gain  Gain=Gp
  INT : Subsystem
  Logical Operator1 : Logic  AllPortsSameDT=off  OutDataTypeStr=boolean
  Logical Operator10 : Logic  Operator=NOT  AllPortsSameDT=off  OutDataTypeStr=boolean
  Logical Operator11 : Logic  Operator=NOT  AllPortsSameDT=off  OutDataTypeStr=boolean
  Logical Operator2 : Logic  AllPortsSameDT=off  OutDataTypeStr=boolean
  Logical Operator3 : Logic  Operator=NOT  AllPortsSameDT=off  OutDataTypeStr=boolean
  Logical_Not1 : Constant  Value=0  SampleTime=-1
  MinMax : MinMax  Inputs=2  InputSameDT=on  SaturateOnIntegerOverflow=on
  MinMax1 : MinMax  Inputs=2  InputSameDT=on  SaturateOnIntegerOverflow=on
  MinMax3 : MinMax  Inputs=2  InputSameDT=on  SaturateOnIntegerOverflow=on
  Product{1..2,23..24} (4 alike) : Product  InputSameDT=on  SaturateOnIntegerOverflow=on  OutDataTypeStr=Inherit: Same as first input
  Relational Operator1 : RelationalOperator  Operator=>  OutDataTypeStr=boolean  InputSameDT=off
  Saturation : Saturate  UpperLimit=1  LowerLimit=0
  Saturation1 : Saturate  UpperLimit=1  LowerLimit=0
  Saturation3 : Saturate  UpperLimit=1  LowerLimit=0
  Sum18 : Sum  Inputs=+--  InputSameDT=on  SaturateOnIntegerOverflow=on  OutDataTypeStr=Inherit: Same as first input
  Sum19 : Sum  Inputs=+--  InputSameDT=on  SaturateOnIntegerOverflow=on  OutDataTypeStr=Inherit: Same as first input
  Sum2 : Sum  Inputs=++++  InputSameDT=on  SaturateOnIntegerOverflow=on  OutDataTypeStr=Inherit: Same as first input
  Sum21 : Sum  InputSameDT=on  SaturateOnIntegerOverflow=on  OutDataTypeStr=Inherit: Same as first input
  Sum3 : Sum  InputSameDT=on  SaturateOnIntegerOverflow=on  OutDataTypeStr=Inherit: Same as first input
  Sum4 : Sum  Inputs=+-----  InputSameDT=on  SaturateOnIntegerOverflow=on  OutDataTypeStr=Inherit: Same as first input
  Sum5 : Sum  InputSameDT=on  SaturateOnIntegerOverflow=on  OutDataTypeStr=Inherit: Same as first input
  Sum6 : Sum  Inputs=-+  InputSameDT=on  SaturateOnIntegerOverflow=on  SampleTime=Ts  OutDataTypeStr=Inherit: Same as first input
  Sum7 : Sum  Inputs=+++  InputSameDT=on  SaturateOnIntegerOverflow=on  OutDataTypeStr=Inherit: Same as first input
  Sum8 : Sum  Inputs=+++  InputSameDT=on  SaturateOnIntegerOverflow=on  OutDataTypeStr=Inherit: Same as first input
  Switch : Switch  Criteria=u2 > Threshold  SaturateOnIntegerOverflow=off  InputSameDT=off
  Switch{1..5} (5 alike) : Switch  Criteria=u2 ~= 0  Threshold=0.5  SaturateOnIntegerOverflow=off  InputSameDT=off
  Terminator : Terminator
  Unit Delay1 : UnitDelay  SampleTime=Ts  HasFrameUpgradeWarning=on
  logic : Subsystem
  IdcPM : Outport  VectorParamsAs1DForOutWhenUnconnected=off
  IdcNM : Outport  Port=2  VectorParamsAs1DForOutWhenUnconnected=off
  Vac : Outport  Port=3  VectorParamsAs1DForOutWhenUnconnected=off
  wires:
  logic/1(Out1) -> Logical Operator1/2
  Relational Operator1/1 -> logic/2(In2)
  [go_lower] -> Terminator/1
  Switch1/1 -> Unit Delay1/1, Vac/1
  Logical Operator2/1 -> [no_pulse]
  Compare To Zero2/1 -> Logical Operator2/2  "1=no-pulse"
  Compare To Zero1/1 -> Logical Operator2/1  "1=no-pulse"
  Sum2/1 -> Compare To Zero2/1
  [q4] -> Sum2/4
  [q3] -> Sum2/3
  [q2] -> Sum2/2
  [q1] -> Sum2/1
  [Vout] -> INT/2(Initial)
  Unit Delay1/1 -> [Vout]
  Iac/1 -> Divide1/1, Divide5/1, Compare To Zero/1, INT/1(u), Gain1/1
  Switch/1 -> Switch1/1
  [q3q4] -> Sum8/3
  [q2q3] -> Sum8/2
  [q1q2] -> Sum8/1
  [i_mid] -> Switch4/1, Switch5/3, Dead Zone1/1
  [i_up] -> Switch2/1, Dead Zone/1, Switch3/3
  [no_pulse] -> Switch5/2
  [no_pulse] -> Switch3/2
  Divide5/1 -> [i_mid]
  [go_neutral] -> Divide5/2
  Switch4/1 -> IdcNM/1
  Dead Zone1/1 -> Switch5/1
  Switch5/1 -> Switch4/3
  [go_upper] -> Divide1/2
  Divide1/1 -> [i_up]
  Sum8/1 -> Compare To Zero1/1
  Divide4/1 -> Sum3/2
  Divide2/1 -> Sum3/1
  [go_neutral] -> Divide4/2
  VNM/1 -> Divide4/1, [VinNM]
  [go_upper] -> Divide2/2
  VPM/1 -> Divide2/1, [VinPM]
  [q2_Vn] -> Sum7/3
  Sum7/1 -> [go_neutral]
  [q3_Vn] -> Sum7/2
  [q2q3] -> Sum7/1
  [q3q4] -> Sum5/1
  [Vn_rem] -> Sum5/2
  [Vp_rem] -> Sum21/2
  Saturation3/1 -> Product1/1, Product2/1
  Data Type Conversion4/1 -> Product2/2
  Product2/1 -> [Vn_rem]
  Data Type Conversion1/1 -> Product1/2
  [current_positive_out] -> Logical Operator11/1, Data Type Conversion4/1
  Logical Operator11/1 -> Data Type Conversion1/1
  Sum4/1 -> Saturation3/1
  Product1/1 -> [Vp_rem]
  [q2_Vn] -> Sum4/6
  [q3_Vn] -> Sum4/5
  [q3q4] -> Sum4/4
  [q2q3] -> Sum4/3
  [q1q2] -> Sum4/2
  Constant1/1 -> Sum4/1
  Sum5/1 -> [go_lower]
  Sum21/1 -> [go_upper]
  [q1q2] -> Sum21/1
  Logical Operator10/1 -> Data Type Conversion3/1
  Data Type Conversion2/1 -> Product24/2
  [current_positive_out] -> Logical Operator10/1
  Sum19/1 -> Saturation1/1
  [q1q2] -> Sum19/3
  Product23/1 -> [q3_Vn]
  [current_positive_out] -> Data Type Conversion2/1
  Saturation/1 -> Product23/1
  Data Type Conversion3/1 -> Product23/2
  Saturation1/1 -> Product24/1
  [q2q3] -> Sum19/2
  Product24/1 -> [q2_Vn]
  [q2] -> Sum19/1
  Sum18/1 -> Saturation/1
  [q3q4] -> Sum18/3
  [q3] -> Sum18/1
  [q2q3] -> Sum18/2
  g4/1 -> MinMax1/2, [q4]
  g2/1 -> [q2], MinMax3/1, MinMax/2
  g3/1 -> MinMax3/2, [q3], MinMax1/1
  g1/1 -> MinMax/1, [q1]
  MinMax1/1 -> [q3q4]
  MinMax/1 -> [q1q2]
  MinMax3/1 -> [q2q3]
  Switch3/1 -> Switch2/3
  Dead Zone/1 -> Switch3/1
  Switch2/1 -> IdcPM/1
  Sum3/1 -> Switch1/3
  Compare To Zero/1 -> logic/1(In1), [current_positive_out]
  [Vout] -> Relational Operator1/2
  [no_pulse] -> Logical Operator1/1
  Logical Operator3/1 -> Divide5/3, Divide1/3
  [VinPM] -> Relational Operator1/1
  INT/1(u_p) -> Sum6/2
  Sum6/1 -> Switch/2, Switch/1
  Logical_Not1/1 -> Switch/3
  Logical Operator1/1 -> Switch2/2, Switch4/2, Switch1/2, Logical Operator3/1, INT/3(en)
  Gain1/1 -> Sum6/1

== system simetranss/Lines/Half-DPL/Simscape ==
  Electrical Reference1 : fl_lib/Electrical/Electrical Elements/Electrical Reference
  PS-S : nesl_utility/PS-Simulink Converter  PhysicalDomain=network_engine_domain  SubClassName=ps_output  LeftPortType=input  RightPortType=output  PseudoPeriodic=off  Frequencies=[]  VectorFormat=1-D array  Unit=V  AffineConversion=off
  Voltage Sensor : fl_lib/Electrical/Electrical Sensors/Voltage Sensor
  V : PMIOPort  Side=Left
  Out : Outport  VectorParamsAs1DForOutWhenUnconnected=off
  wires:
  PS-S/1 -> Out/1  "voltage"
  connections:
  PS-S/LConn1 -- Voltage Sensor/RConn1
  V/RConn1 -- Voltage Sensor/LConn1
  Electrical Reference1/LConn1 -- Voltage Sensor/RConn2

== system simetranss/Lines/Half-DPL/Simscape1 ==
  Electrical Reference1 : fl_lib/Electrical/Electrical Elements/Electrical Reference
  PS-S : nesl_utility/PS-Simulink Converter  PhysicalDomain=network_engine_domain  SubClassName=ps_output  LeftPortType=input  RightPortType=output  PseudoPeriodic=off  Frequencies=[]  VectorFormat=1-D array  Unit=V  AffineConversion=off
  Voltage Sensor : fl_lib/Electrical/Electrical Sensors/Voltage Sensor
  V : PMIOPort  Side=Left
  Out : Outport  VectorParamsAs1DForOutWhenUnconnected=off
  wires:
  PS-S/1 -> Out/1  "voltage"
  connections:
  Electrical Reference1/LConn1 -- Voltage Sensor/RConn2
  V/RConn1 -- Voltage Sensor/LConn1
  PS-S/LConn1 -- Voltage Sensor/RConn1

== system simetranss/Lines/Half-DPL/Simscape2 ==
  Electrical Reference1 : fl_lib/Electrical/Electrical Elements/Electrical Reference
  PS-S : nesl_utility/PS-Simulink Converter  PhysicalDomain=network_engine_domain  SubClassName=ps_output  LeftPortType=input  RightPortType=output  PseudoPeriodic=off  Frequencies=[]  VectorFormat=1-D array  Unit=V  AffineConversion=off
  Voltage Sensor : fl_lib/Electrical/Electrical Sensors/Voltage Sensor
  V : PMIOPort  Side=Left
  Out : Outport  VectorParamsAs1DForOutWhenUnconnected=off
  wires:
  PS-S/1 -> Out/1  "voltage"
  connections:
  PS-S/LConn1 -- Voltage Sensor/RConn1
  V/RConn1 -- Voltage Sensor/LConn1
  Electrical Reference1/LConn1 -- Voltage Sensor/RConn2

== system simetranss/Lines/Half-DPL/Voltage Source ==
  I : Inport
  Controlled Current Source1 : fl_lib/Electrical/Electrical Sources/Controlled Current Source
  Simulink-PS Converter : nesl_utility/Simulink-PS Converter  PhysicalDomain=network_engine_domain  SubClassName=ps_input  LeftPortType=input  RightPortType=output  PseudoPeriodic=off  Frequencies=[]  NoiseDistribution=none  NoiseParameters=[]  Unit=1  AffineConversion=off  FilteringAndDerivatives=zero  SimscapeFilterOrder=1  InputFilterTimeConstant=.001  UdotUserProvided=0
  + : PMIOPort  Side=Right
  - : PMIOPort  Port=2  Side=Right
  wires:
  I/1 -> Simulink-PS Converter/1
  connections:
  Controlled Current Source1/RConn1 -- Simulink-PS Converter/RConn1
  Controlled Current Source1/RConn2 -- -/RConn1
  Controlled Current Source1/LConn1 -- +/RConn1

== system simetranss/Lines/Half-DPL/Voltage Source1 ==
  I : Inport
  Controlled Current Source1 : fl_lib/Electrical/Electrical Sources/Controlled Current Source
  Simulink-PS Converter : nesl_utility/Simulink-PS Converter  PhysicalDomain=network_engine_domain  SubClassName=ps_input  LeftPortType=input  RightPortType=output  PseudoPeriodic=off  Frequencies=[]  NoiseDistribution=none  NoiseParameters=[]  Unit=1  AffineConversion=off  FilteringAndDerivatives=zero  SimscapeFilterOrder=1  InputFilterTimeConstant=.001  UdotUserProvided=0
  + : PMIOPort  Side=Right
  - : PMIOPort  Port=2  Side=Right
  wires:
  I/1 -> Simulink-PS Converter/1
  connections:
  Controlled Current Source1/LConn1 -- +/RConn1
  Controlled Current Source1/RConn2 -- -/RConn1
  Controlled Current Source1/RConn1 -- Simulink-PS Converter/RConn1

== system simetranss/Lines/Half-DPL/Voltage Source2 ==
  I : Inport
  Controlled Current Source1 : fl_lib/Electrical/Electrical Sources/Controlled Current Source
  Simulink-PS Converter : nesl_utility/Simulink-PS Converter  PhysicalDomain=network_engine_domain  SubClassName=ps_input  LeftPortType=input  RightPortType=output  PseudoPeriodic=off  Frequencies=[]  NoiseDistribution=none  NoiseParameters=[]  Unit=1  AffineConversion=off  FilteringAndDerivatives=zero  SimscapeFilterOrder=1  InputFilterTimeConstant=.001  UdotUserProvided=0
  + : PMIOPort  Side=Right
  - : PMIOPort  Port=2  Side=Right
  wires:
  I/1 -> Simulink-PS Converter/1
  connections:
  Controlled Current Source1/RConn1 -- Simulink-PS Converter/RConn1
  Controlled Current Source1/RConn2 -- -/RConn1
  Controlled Current Source1/LConn1 -- +/RConn1

== system simetranss/Lines/Half-DPL/dplmodel ==
  v : Inport
  hist_in : Inport  Port=2
  (1+h)/Z : Gain  Gain=(1+h)./(Zm+Rt4)  SaturateOnIntegerOverflow=on  OutDataTypeStr=Inherit: Same as input  ParamDataTypeStr=Inherit: Same as input
  Gain4 : Gain  Gain=(1+h)/2  SaturateOnIntegerOverflow=on  OutDataTypeStr=Inherit: Same as input  ParamDataTypeStr=Inherit: Same as input
  Gain6 : Gain  Gain=(1-h)/2  SaturateOnIntegerOverflow=on  OutDataTypeStr=Inherit: Same as input  ParamDataTypeStr=Inherit: Same as input
  Gain9 : Gain  Gain=h  SaturateOnIntegerOverflow=on  OutDataTypeStr=Inherit: Same as input  ParamDataTypeStr=Inherit: Same as input
  Matrix Gain1 : StateSpace  A=[]  B=[]  C=[]  D=K  InitialCondition=0  mask(Matrix Gain){K=Ti'}
      mask prompts: K "Gain matrix:"
      mask help: Matrix Gain.
      mask Help: Multiplies input vector by entered matrix to produce output vector (y=Au).
      mask Display: disp('K')
  Matrix Gain2 : StateSpace  A=[]  B=[]  C=[]  D=K  InitialCondition=0  mask(Matrix Gain){K=Ti}
      mask prompts: K "Gain matrix:"
      mask help: Matrix Gain.
      mask Help: Multiplies input vector by entered matrix to produce output vector (y=Au).
      mask Display: disp('K')
  Subsystem : Subsystem
  Sum1 : Sum  Inputs=-+  InputSameDT=on  SaturateOnIntegerOverflow=on  OutDataTypeStr=Inherit: Same as first input
  Sum3 : Sum  InputSameDT=on  SaturateOnIntegerOverflow=on  OutDataTypeStr=Inherit: Same as first input
  i : Outport  InitialOutput=0  VectorParamsAs1DForOutWhenUnconnected=off
  hist_out : Outport  Port=2  VectorParamsAs1DForOutWhenUnconnected=off
  wires:
  Matrix Gain2/1 -> i/1
  Matrix Gain1/1 -> (1+h)/Z/1
  Gain4/1 -> hist_out/1
  Gain9/1 -> Sum1/1
  Sum3/1 -> Matrix Gain2/1, Gain9/1
  (1+h)/Z/1 -> Sum1/2
  v/1 -> Matrix Gain1/1
  Gain6/1 -> Sum3/1
  hist_in/1 -> Sum3/2
  Subsystem/1(Out1) -> Gain4/1, Gain6/1
  Sum1/1 -> Subsystem/1(In1)

== system simetranss/Lines/Half-DPL1ph/Simscape ==
  Electrical Reference1 : fl_lib/Electrical/Electrical Elements/Electrical Reference
  PS-S : nesl_utility/PS-Simulink Converter  PhysicalDomain=network_engine_domain  SubClassName=ps_output  LeftPortType=input  RightPortType=output  PseudoPeriodic=off  Frequencies=[]  VectorFormat=1-D array  Unit=V  AffineConversion=off
  Voltage Sensor : fl_lib/Electrical/Electrical Sensors/Voltage Sensor
  V : PMIOPort  Side=Left
  Out : Outport  VectorParamsAs1DForOutWhenUnconnected=off
  wires:
  PS-S/1 -> Out/1  "voltage"
  connections:
  PS-S/LConn1 -- Voltage Sensor/RConn1
  V/RConn1 -- Voltage Sensor/LConn1
  Electrical Reference1/LConn1 -- Voltage Sensor/RConn2

== system simetranss/Lines/Half-DPL1ph/Voltage Source ==
  I : Inport
  Controlled Current Source1 : fl_lib/Electrical/Electrical Sources/Controlled Current Source
  Simulink-PS Converter : nesl_utility/Simulink-PS Converter  PhysicalDomain=network_engine_domain  SubClassName=ps_input  LeftPortType=input  RightPortType=output  PseudoPeriodic=off  Frequencies=[]  NoiseDistribution=none  NoiseParameters=[]  Unit=1  AffineConversion=off  FilteringAndDerivatives=zero  SimscapeFilterOrder=1  InputFilterTimeConstant=.001  UdotUserProvided=0
  + : PMIOPort  Side=Right
  - : PMIOPort  Port=2  Side=Right
  wires:
  I/1 -> Simulink-PS Converter/1
  connections:
  Controlled Current Source1/RConn1 -- Simulink-PS Converter/RConn1
  Controlled Current Source1/RConn2 -- -/RConn1
  Controlled Current Source1/LConn1 -- +/RConn1

== system simetranss/Lines/Half-DPL1ph/dplmodel ==
  v : Inport
  hist_in : Inport  Port=2
  (1+h)/Z : Gain  Gain=(1+h)./(Zm+Rt4)  SaturateOnIntegerOverflow=on  OutDataTypeStr=Inherit: Same as input  ParamDataTypeStr=Inherit: Same as input
  Gain4 : Gain  Gain=(1+h)/2  SaturateOnIntegerOverflow=on  OutDataTypeStr=Inherit: Same as input  ParamDataTypeStr=Inherit: Same as input
  Gain6 : Gain  Gain=(1-h)/2  SaturateOnIntegerOverflow=on  OutDataTypeStr=Inherit: Same as input  ParamDataTypeStr=Inherit: Same as input
  Gain9 : Gain  Gain=h  SaturateOnIntegerOverflow=on  OutDataTypeStr=Inherit: Same as input  ParamDataTypeStr=Inherit: Same as input
  Sum1 : Sum  Inputs=-+  InputSameDT=on  SaturateOnIntegerOverflow=on  OutDataTypeStr=Inherit: Same as first input
  Sum3 : Sum  InputSameDT=on  SaturateOnIntegerOverflow=on  OutDataTypeStr=Inherit: Same as first input
  derlay : Subsystem
  i : Outport  InitialOutput=0  VectorParamsAs1DForOutWhenUnconnected=off
  hist_out : Outport  Port=2  VectorParamsAs1DForOutWhenUnconnected=off
  wires:
  Sum3/1 -> i/1, Gain9/1
  v/1 -> (1+h)/Z/1
  Gain4/1 -> hist_out/1
  Gain9/1 -> Sum1/1
  (1+h)/Z/1 -> Sum1/2
  Gain6/1 -> Sum3/1
  hist_in/1 -> Sum3/2
  derlay/1(Out1) -> Gain4/1, Gain6/1
  Sum1/1 -> derlay/1(In1)

== system simetranss/Machines/MATE 6//4 SRM/Pos_sensor ==
  w : Inport
  Constant : Constant  Value=pi/2
  Discrete-Time Integrator : DiscreteIntegrator  InitialCondition=init_rotor_pos*pi/180  SampleTime=Ts  ICPrevOutput=DiscIntNeverNeededParam  ICPrevScaledInput=DiscIntNeverNeededParam
  Math Function : Math  Operator=mod  SignedPower=on
  angle : Outport  VectorParamsAs1DForOutWhenUnconnected=off
  wires:
  Math Function/1 -> angle/1
  Constant/1 -> Math Function/2
  Discrete-Time Integrator/1 -> Math Function/1
  w/1 -> Discrete-Time Integrator/1

== system simetranss/Machines/MATE Induction Machine/1 step prediction+2step averaging ==
  In1 : Inport
  Gain1 : Gain  Gain=0.5
  Gain2 : Gain  Gain=2
  Gain3 : Gain  Gain=-1
  Sum1 : Sum  SaturateOnIntegerOverflow=on
  Sum5 : Sum  SaturateOnIntegerOverflow=on
  Unit Delay1 : UnitDelay  SampleTime=Ts  HasFrameUpgradeWarning=on
  Out1 : Outport  VectorParamsAs1DForOutWhenUnconnected=off
  wires:
  In1/1 -> Sum1/2, Unit Delay1/1, Gain2/1
  Gain3/1 -> Sum5/2
  Gain2/1 -> Sum5/1
  Unit Delay1/1 -> Gain3/1
  Sum5/1 -> Sum1/1
  Sum1/1 -> Gain1/1
  Gain1/1 -> Out1/1

== system simetranss/Machines/MATE Induction Machine/Discretize (rotor Frame) ==
  Ac : Inport
  Bc : Inport  Port=2
  Cc : Inport  Port=3
  be : Inport  Port=4
  Enable : EnablePort
  2 euler factor : Gain  Gain=2  SaturateOnIntegerOverflow=on  OutDataTypeStr=Inherit: Same as input  ParamDataTypeStr=Inherit: Same as input
  Product1 : Product  Multiplication=Matrix(*)  SaturateOnIntegerOverflow=on  OutDataTypeStr=Inherit: Same as first input
  Product2 : Product  Multiplication=Matrix(*)  SaturateOnIntegerOverflow=on  OutDataTypeStr=Inherit: Same as first input
  Product4 : Product  Multiplication=Matrix(*)  SaturateOnIntegerOverflow=on  OutDataTypeStr=Inherit: Same as first input
  Sum1 : Sum  Inputs=+-  SaturateOnIntegerOverflow=on
  Sum2 : Sum  Inputs=2  SaturateOnIntegerOverflow=on
  Sum4 : Sum  Inputs=-+  SaturateOnIntegerOverflow=on
  Sum5 : Sum  SaturateOnIntegerOverflow=on
  Ts/2 : Gain  Gain=Ts/2  SaturateOnIntegerOverflow=on  OutDataTypeStr=Inherit: Same as input  ParamDataTypeStr=Inherit: Same as input
  inversion : Product  Inputs=/  Multiplication=Matrix(*)  RndMeth=Zero
  mult1 : Product
  mult2 : Product
  mult3 : Product
  trapeze has Ts/2 factor on B : Gain  Gain=Ts/2  SaturateOnIntegerOverflow=on  OutDataTypeStr=Inherit: Same as input  ParamDataTypeStr=Inherit: Same as input
  u1 : Constant
  u2 : Constant
  u3 : Constant  Value=eye(4,4)*Ts/2
  u5 : Constant  Value=eye(4,4)
  Ad : Outport  VectorParamsAs1DForOutWhenUnconnected=off
  Bd : Outport  Port=2  VectorParamsAs1DForOutWhenUnconnected=off
  Cd : Outport  Port=3  VectorParamsAs1DForOutWhenUnconnected=off
  bet : Outport  Port=4  VectorParamsAs1DForOutWhenUnconnected=off
  Bdspeedterm : Outport  Port=5  VectorParamsAs1DForOutWhenUnconnected=off
  wires:
  2 euler factor/1 -> Bdspeedterm/1
  Product2/1 -> 2 euler factor/1
  Sum2/1 -> mult2/2, mult1/2
  u3/1 -> Product2/2
  mult2/1 -> Product1/2
  Sum4/1 -> bet/1, mult3/2
  mult3/1 -> Sum5/2
  mult1/1 -> mult3/1, Sum1/2
  u1/1 -> Sum4/2
  be/1 -> Sum4/1, Sum2/2
  u2/1 -> Sum2/1
  Bc/1 -> trapeze has Ts/2 factor on B/1
  Cc/1 -> Cd/1
  inversion/1 -> Product4/1, Product2/1, Product1/1  "inv(I4-Ts/2*A)"
  trapeze has Ts/2 factor on B/1 -> mult2/1
  Ts/2/1 -> mult1/1
  Product4/1 -> Ad/1
  u5/1 -> Sum5/1, Sum1/1
  Sum5/1 -> Product4/2
  Product1/1 -> Bd/1
  Ac/1 -> Ts/2/1
  Sum1/1 -> inversion/1

== system simetranss/Machines/MATE Induction Machine/Discretize(fixed frame) ==
  Cc : Inport
  be : Inport  Port=2
  Enable : EnablePort
  Sum4 : Sum  Inputs=-+  SaturateOnIntegerOverflow=on
  u1 : Constant
  u3 : Constant  Value=Bdspeed
  u4 : Constant  Value=Ad
  u6 : Constant  Value=Bd
  Ad : Outport  VectorParamsAs1DForOutWhenUnconnected=off
  Bd : Outport  Port=2  VectorParamsAs1DForOutWhenUnconnected=off
  Cd : Outport  Port=3  VectorParamsAs1DForOutWhenUnconnected=off
  bet : Outport  Port=4  VectorParamsAs1DForOutWhenUnconnected=off
  Bdspeedterm : Outport  Port=5  VectorParamsAs1DForOutWhenUnconnected=off
  wires:
  u4/1 -> Ad/1
  u6/1 -> Bd/1
  Cc/1 -> Cd/1
  be/1 -> Sum4/1
  u1/1 -> Sum4/2
  Sum4/1 -> bet/1
  u3/1 -> Bdspeedterm/1

== system simetranss/Machines/MATE Induction Machine/MATE ==
  note: D=[] for IM
  Ad : Inport
  Bd : Inport  Port=2
  Cd : Inport  Port=3
  u : Inport  Port=4
  bet : Inport  Port=5
  Bd_sp_term : Inport  Port=6
  u_speedterm : Inport  Port=7
  Gain : Gain
  Product{2..3,5..6,8} (5 alike) : Product  Multiplication=Matrix(*)  SaturateOnIntegerOverflow=on  OutDataTypeStr=Inherit: Same as first input
  Sum2 : Sum  Inputs=+++  SaturateOnIntegerOverflow=on
  Sum3 : Sum  SaturateOnIntegerOverflow=on
  mult2 : Product
  z-1 : UnitDelay  SampleTime=Ts  HasFrameUpgradeWarning=on
  z-2 : UnitDelay  SampleTime=Ts  HasFrameUpgradeWarning=on
  Y : Outport  VectorParamsAs1DForOutWhenUnconnected=off
  Ihist : Outport  Port=2  VectorParamsAs1DForOutWhenUnconnected=off
  phi : Outport  Port=3  VectorParamsAs1DForOutWhenUnconnected=off
  wires:
  z-2/1 -> Product5/1
  Sum3/1 -> Product3/2, phi/1  "new_x"
  mult2/1 -> Sum2/2
  Product8/1 -> Sum2/3
  u_speedterm/1 -> Product8/2
  Bd_sp_term/1 -> Product8/1
  bet/1 -> mult2/2
  z-1/1 -> Sum3/1
  Gain/1 -> Ihist/1
  u/1 -> Product5/2
  Bd/1 -> z-2/1, Product2/2
  Ad/1 -> Product3/1
  Product6/1 -> Gain/1  "C*(Ad*phi_n+Bd*u_n)"
  Sum2/1 -> Product6/2, z-1/1  "Ad*phi_n+Bd*u_n"
  Product3/1 -> Sum2/1
  Product5/1 -> mult2/1, Sum3/2
  Product2/1 -> Y/1  "C*B+D"
  Cd/1 -> Product6/1, Product2/1
